simulink model "SML_SSE_RL"  (R2015a)
settings: Solver=ode4  SolverMode=MultiTasking  StartTime=0.0  StopTime=inf  FixedStep=BKIN_STEP_TIME  RelTol=1e-3
StartFcn:
  |  warndlg('Dexterit-E models cannot run under simulation. Please compile your model and run it from within Dexterit-E.');set_param(bdroot,'SimulationCommand','stop')
model workspace (MAT data in the model file):
  col_x = 1
  col_y = 2
  RADIUS_VIS = 3
  COLOR_INIT = 6
  BKIN_STEP_TIME = 0.00025
  E_END_TRIAL = 20
  STROKE_WIDTH = 8
  K_ROBOT_RAMP_TIME = 1
  E_ENABLED_CONTROLLER = 31
  K_TIME_TO_START = 4
  BKIN_KINEMATIC_FRAME_SIZE = 400
  E_NO_EVENT = 0
  STARTTARGET_COL = 1
  MOVE_TIME_COL = 3
  MOVE_XVEL_COL = 4
  MOVE_YVEL_COL = 5
  E_INIT_TRIAL = 1
  E_MOVE_TO_START = 2
  E_AT_START = 4
  E_PASSIVE_HOLD_AT_START = 6
  E_MOVE_TO_END = 8
  COLOR_SELECT = 7
  ACTORPAS_COL = 6
  E_ACTIVE_HOLD_AT_START = 7
  CHANNEL_WIDTH = 1
  WALL_WIDTH = 2
  WALL_STIFFNESS = 3
  WALL_VISCOSITY = 4
  PROBE_COL = 8
  K_TIME_HOLD_START = 5
  E_ENABLE_BUTTONS = 46
  E_DISABLE_BUTTONS = 47
  LABEL_1 = 3
  RESPONSE_AHEAD = 4
  RESPONSE_BEHIND = 5
  B_LABEL_1 = 3
  B_AHEAD = 4
  B_BEHIND = 5
  DYNOREND_COL = 7
  E_REPEAT_TRIAL_FLAG = 35
  END_TARGET_COL = 2
  HEIGHT_VIS = 4
  WIDTH_VIS = 5
  E_TOO_FAST = 11
  E_TOO_SLOW = 12
  PROBE_SHIFT_COL = 9
  K_TIME_PROBE_HOLD = 3
  E_AT_END_TARGET = 10
  K_DELAY_POSTTRIAL = 2
  LABEL_TEXT = 9
  LABEL_HEIGHT = 10
  E_FINISH_MOVE = 49
  E_HIT_PROBE = 48
  E_TEST_1 = 50
  E_JUST_RIGHT = 51
undefined symbols (not defined in the file): slselsubs
libraries: slrtlib x5, KINARM_loads x4, Video x4, General x3, KINARM_general x2, simulink x1, xpcnilib x1
(part 2 of 2)

== matlab function SML_SSE_RL/Force Channel1/Calculate force channel (wall)  ==
  data: target1 input; forces output; target2 input; active_arm input; hand_position input; hand_velocity input; secondary_encoders_used input; loadTable input; enable_forces input
function forces = forceChannel(target1, target2, active_arm, hand_position, hand_velocity, secondary_encoders_used, loadTable, enable_forces)

	persistent lastForcesEnabledValue forceEnableTime clockCycle outsideChannel lastHandPosition;
	
	if isempty(lastForcesEnabledValue), lastForcesEnabledValue = 0;		end
	if isempty(forceEnableTime),        forceEnableTime = 1;			end
	if isempty(clockCycle),				clockCycle = 0;					end
	if isempty(outsideChannel),			outsideChannel = 0;				end
	if isempty(lastHandPosition),		lastHandPosition = zeros(1,2);	end


	%we need to keep track of the time so we can safely ramp up forces when 
	%the trial starts.
	clockCycle = clockCycle + 1;
	if lastForcesEnabledValue == 0 && enable_forces == 1
		forceEnableTime = clockCycle;
	end

	lastForcesEnabledValue = enable_forces;

	%start out assuming we will apply no forces.
	forces = zeros(1, 4);

    channelWidthM = abs((loadTable(1) * 0.01) / 2.0);%get the width of the zero force zone and convert to meters
	wallWidthM = abs(loadTable(2) * 0.01);			%get the width of the wall where forces cut out and convert to meters.
%     if secondary_encoders_used == 0
%         % No secondary encoders
%     	wallStiffness = abs(loadTable(3));				%in N/m
%     	viscosity = -abs(loadTable(4));					%in N/(m/s)
%     else
        % With secondary encoders
    	wallStiffness = abs(loadTable(3));				%in N/m
    	viscosity = -abs(loadTable(4));					%in N/(m/s)
%     end

	xHand=hand_position(1);		%(m)
	yHand=hand_position(2);		%(m)

	%get the target positions and convert them to meters.
	x1 = (-20) * 0.01; 
    %y1 = target1-(loadTable(1)/2)* 0.01;
	y1 = target1* 0.01;   %offset for half of the channel zero force width... puts wall at center of probe instead of at radius.
	x2 = (20) * 0.01;                       %target 2 is projected from target1 and the desired start velocities
	%y2 = target2-(loadTable(1)/2) * 0.01;
    y2 = target2 * 0.01;

	%http://www.codeguru.com/forum/showthread.php?threadid=194400
	%This calculations gives us the distance away from the line we are now.
	distToLine = abs(((x2 - x1)*(y1-yHand)) - ((x1 - xHand)*(y2-y1))) / sqrt( (x2 - x1)^2 + (y2 - y1)^2 );

	HXVEL = hand_velocity(1);
	HYVEL = hand_velocity(2);
	viscosityX = HXVEL * viscosity;
	viscosityY = HYVEL * viscosity;

	%we only ever want to provide a viscous load perpendicular to
	%the force channel. This viscous force will be used to dampen
	%any instability.
	if (x2 == x1) %infinite slope
		viscosityY = 0;	
	elseif (y2 == y1) %0 slope
		viscosityX = 0;
	else
		m = (y2 - y1) / (x2 - x1);
		perpM = -(1/m);	

		%we need to scale the viscous load to only the components
		%that are perpendicular to the line. To do that we find the 
		%projection of the velocity vecotor on a line perpendicular to the
		%force channel
		perpVect = [1 perpM];
		perpUnitVector = perpVect / norm(perpVect);

		%this finds the projection of the vector perpendicular to the channel
		dotProduct = dot([viscosityX viscosityY], perpUnitVector);
		scaledForces = dotProduct * perpUnitVector;

		viscosityX = scaledForces(1);
		viscosityY = scaledForces(2);
	end

	%forces 1,2 are for right arm, 3,4 are for left
	addIdx = 0;
	if active_arm == 2
		addIdx = 2;
	end

	% if we are outside the force wall we need to make sure we don't turn it
	%back on until we are in the channel. Otherwise it's quite jarring to be pulled in.
	if distToLine > (wallWidthM + channelWidthM)
		outsideChannel = 1;
		return
	elseif enable_forces == 0
		return	
	%if we are in the force channel we still need to viscous loads to aid in stability
	%if we are bouncing between the walls. 
	elseif distToLine < channelWidthM 
		outsideChannel = 0; %we're in the channel, so we can turn forces back on if they were off.
		return
	elseif outsideChannel == 1    
		%If we were outside the wall then forces are all off. We only want to turn
		%forces back on if the hand has crossed the line of the force channel, that way
		%you are not pushed into the channel, it only feels like you hit a wall.
		%By looking at the previous hand position and the current hand position
		%we can see if that line segment crosses the channel line, in which case we can
		%turn the forces back on.
		if doLinesIntersect([x1 y1], [x2 y2], [xHand yHand], lastHandPosition) == 1
			outsideChannel = 0;
		else
			return
		end
	end

	distIntoWall = distToLine - channelWidthM;

	if (x2 == x1) %all force wille be in x direction
		y = 0;
		if xHand < x1
			x = distIntoWall;
		else
			x = -distIntoWall;
		end
	elseif (y2 == y1) %all force will be in Y direction
		x = 0;
		if yHand < y1
			y = distIntoWall;
		else
			y = -distIntoWall;
		end	
	else
		%we need to find out how far off the line in X and Y we are in meters so 
		%we can properly convert the wall stiffness in N/m to a force.
		m = (y2 - y1) / (x2 - x1);
		b = y1 - (m * x1);

		perpM = -(1/m);	
		perpB = yHand - (perpM * xHand);

		xIntersect = (b - perpB) / (perpM - m);
		yIntersect = (m * xIntersect) + b;

		%x and y are converted to distances in meters from the center line
		x = xIntersect - xHand;
		y = yIntersect - yHand;

		%take the distances from center and convert to a unit vector,
		%then multiply by the distance to where the forces start
		%this gives us a clean number to use when calculating wall force.
		x = (x / sqrt(x^2 + y^2)) * distIntoWall;
		y = (y / sqrt(x^2 + y^2)) * distIntoWall;
	end

	%we don't want to just shut off the forces, we need to ramp them down
	%somewhat. This finds out how far into the wall we are and allows us
	%to ramp down the forces over the last X% of the wll.
	forceRampDownZoneSizePercent = 0.9; %start ramping down the forces in the last 25% of the wall
	forceMaxEndLocInWallM = forceRampDownZoneSizePercent * wallWidthM;
	distanceIntoWall = distToLine - channelWidthM;
	scaleWallForce = 1; %assume we can run at full calculated wall force

	if distanceIntoWall > forceMaxEndLocInWallM   %we are in the ramp down zone
		distIntoRampDownZone = distanceIntoWall - forceMaxEndLocInWallM;
		rampDownZoneWidth = wallWidthM  - forceMaxEndLocInWallM;
		scaleWallForce = (rampDownZoneWidth - distIntoRampDownZone) / rampDownZoneWidth;
	end

	%within the first 1.5 seconds of the trial we don't wan to jar anyone
	%this ramps the forces up slowly so you get a gentle nudge into
	%the force channel, not a violent jerk.
	timeDelta = clockCycle - forceEnableTime;
	timeScaling = 1;
	if (timeDelta < 1500)
		timeScaling = timeDelta / 1500.0;
	end

	%the final forces will be wall force + viscous.
	forces(addIdx + 1) = (wallStiffness * scaleWallForce * timeScaling * x) + viscosityX;
	forces(addIdx + 2) = (wallStiffness * scaleWallForce  * timeScaling * y) + viscosityY;

	lastHandPosition(1) = xHand;
	lastHandPosition(2) = yHand;
end

function bIntersect = doLinesIntersect(Ap1, Ap2, Bp1, Bp2)
    %This method for finding out if 2 lines segements intersect comes from:
    %http://stackoverflow.com/questions/563198/how-do-you-detect-where-two-line-segments-intersect
   	e = Ap2-Ap1;
    f = Bp2-Bp1;
    p = [-e(2) e(1)];
    h = dot((Ap1 - Bp1), p) / dot (f, p);
    
    if h >=0 && h <= 1
        bIntersect = 1;
    else
        bIntersect = 0;
    end
end

== matlab function SML_SSE_RL/Play Sound/Play sound over and over ==
  data: tone input; output output; Hz500 input; Hz800 input; Hz1200 input
function output = fcn(tone,Hz500,Hz800,Hz1200)
%#codegen

persistent t last_tone_state
if isempty(t), t = 0; end
if isempty(last_tone_state), last_tone_state = 0; end

trigger = last_tone_state ~= tone;
if trigger > 0
    last_tone_state = tone;
end

output = 0;		% default
if t == 0 && trigger > 0
	% start the playing of the sound.
	t = t + 1;
end

if tone == 1
    data = Hz500;
elseif tone == 2
    data = Hz800;
elseif tone == 3
    data = Hz1200;
else 
    t = 0;
    data = 0;
end

if t > 0
	output = data(t);
	if t == length(data)
		t = 0;
	else
		t = t + 1;
	end
end

== matlab function SML_SSE_RL/Force Channel/Calculate force channel ==
  data: target1 input; forces output; target2 input; xIdx input; yIdx input; active_arm input; hand_position input; hand_velocity input; secondary_encoders_used input; loadTable input; enable_forces input
function forces = forceChannel(target1, target2, xIdx, yIdx, active_arm, hand_position, hand_velocity, secondary_encoders_used, loadTable, enable_forces)

	persistent lastForcesEnabledValue forceEnableTime clockCycle outsideChannel lastHandPosition;
	
	if isempty(lastForcesEnabledValue), lastForcesEnabledValue = 0;		end
	if isempty(forceEnableTime),        forceEnableTime = 1;			end
	if isempty(clockCycle),				clockCycle = 0;					end
	if isempty(outsideChannel),			outsideChannel = 0;				end
	if isempty(lastHandPosition),		lastHandPosition = zeros(1,2);	end


	%we need to keep track of the time so we can safely ramp up forces when 
	%the trial starts.
	clockCycle = clockCycle + 1;
	if lastForcesEnabledValue == 0 && enable_forces == 1
		forceEnableTime = clockCycle;
	end

	lastForcesEnabledValue = enable_forces;

	%start out assuming we will apply no forces.
	forces = zeros(1, 4);

    channelWidthM = abs((loadTable(1) * 0.01) / 2.0);%get the width of the zero force zone and convert to meters
	wallWidthM = abs(loadTable(2) * 0.01);			%get the width of the wall where forces cut out and convert to meters.
%     if secondary_encoders_used == 0
%         % No secondary encoders
%     	wallStiffness = abs(loadTable(3));				%in N/m
%     	viscosity = -abs(loadTable(4));					%in N/(m/s)
%     else
        % With secondary encoders
    	wallStiffness = abs(loadTable(3));				%in N/m
    	viscosity = -abs(loadTable(4));					%in N/(m/s)
%     end

	xHand=hand_position(1);		%(m)
	yHand=hand_position(2);		%(m)

	%get the target positions and convert them to meters.
	x1 = target1(xIdx) * 0.01;
	y1 = target1(yIdx) * 0.01;
	x2 = target2(1) * 0.01;  %target 2 is projected from target1 and the desired start velocities
	y2 = target2(2) * 0.01;

	%http://www.codeguru.com/forum/showthread.php?threadid=194400
	%This calculations gives us the distance away from the line we are now.
	distToLine = abs(((x2 - x1)*(y1-yHand)) - ((x1 - xHand)*(y2-y1))) / sqrt( (x2 - x1)^2 + (y2 - y1)^2 );

	HXVEL = hand_velocity(1);
	HYVEL = hand_velocity(2);
	viscosityX = HXVEL * viscosity;
	viscosityY = HYVEL * viscosity;

	%we only ever want to provide a viscous load perpendicular to
	%the force channel. This viscous force will be used to dampen
	%any instability.
	if (x2 == x1) %infinite slope
		viscosityY = 0;	
	elseif (y2 == y1) %0 slope
		viscosityX = 0;
	else
		m = (y2 - y1) / (x2 - x1);
		perpM = -(1/m);	

		%we need to scale the viscous load to only the components
		%that are perpendicular to the line. To do that we find the 
		%projection of the velocity vecotor on a line perpendicular to the
		%force channel
		perpVect = [1 perpM];
		perpUnitVector = perpVect / norm(perpVect);

		%this finds the projection of the vector perpendicular to the channel
		dotProduct = dot([viscosityX viscosityY], perpUnitVector);
		scaledForces = dotProduct * perpUnitVector;

		viscosityX = scaledForces(1);
		viscosityY = scaledForces(2);
	end

	%forces 1,2 are for right arm, 3,4 are for left
	addIdx = 0;
	if active_arm == 2
		addIdx = 2;
	end

	% if we are outside the force wall we need to make sure we don't turn it
	%back on until we are in the channel. Otherwise it's quite jarring to be pulled in.
	if distToLine > (wallWidthM + channelWidthM)
		outsideChannel = 1;
		return
	elseif enable_forces == 0
		return	
	%if we are in the force channel we still need to viscous loads to aid in stability
	%if we are bouncing between the walls. 
	elseif distToLine < channelWidthM 
		outsideChannel = 0; %we're in the channel, so we can turn forces back on if they were off.
		return
	elseif outsideChannel == 1    
		%If we were outside the wall then forces are all off. We only want to turn
		%forces back on if the hand has crossed the line of the force channel, that way
		%you are not pushed into the channel, it only feels like you hit a wall.
		%By looking at the previous hand position and the current hand position
		%we can see if that line segment crosses the channel line, in which case we can
		%turn the forces back on.
		if doLinesIntersect([x1 y1], [x2 y2], [xHand yHand], lastHandPosition) == 1
			outsideChannel = 0;
		else
			return
		end
	end

	distIntoWall = distToLine - channelWidthM;

	if (x2 == x1) %all force wille be in x direction
		y = 0;
		if xHand < x1
			x = distIntoWall;
		else
			x = -distIntoWall;
		end
	elseif (y2 == y1) %all force will be in Y direction
		x = 0;
		if yHand < y1
			y = distIntoWall;
		else
			y = -distIntoWall;
		end	
	else
		%we need to find out how far off the line in X and Y we are in meters so 
		%we can properly convert the wall stiffness in N/m to a force.
		m = (y2 - y1) / (x2 - x1);
		b = y1 - (m * x1);

		perpM = -(1/m);	
		perpB = yHand - (perpM * xHand);

		xIntersect = (b - perpB) / (perpM - m);
		yIntersect = (m * xIntersect) + b;

		%x and y are converted to distances in meters from the center line
		x = xIntersect - xHand;
		y = yIntersect - yHand;

		%take the distances from center and convert to a unit vector,
		%then multiply by the distance to where the forces start
		%this gives us a clean number to use when calculating wall force.
		x = (x / sqrt(x^2 + y^2)) * distIntoWall;
		y = (y / sqrt(x^2 + y^2)) * distIntoWall;
	end

	%we don't want to just shut off the forces, we need to ramp them down
	%somewhat. This finds out how far into the wall we are and allows us
	%to ramp down the forces over the last X% of the wll.
	forceRampDownZoneSizePercent = 0.9; %start ramping down the forces in the last 25% of the wall
	forceMaxEndLocInWallM = forceRampDownZoneSizePercent * wallWidthM;
	distanceIntoWall = distToLine - channelWidthM;
	scaleWallForce = 1; %assume we can run at full calculated wall force

	if distanceIntoWall > forceMaxEndLocInWallM   %we are in the ramp down zone
		distIntoRampDownZone = distanceIntoWall - forceMaxEndLocInWallM;
		rampDownZoneWidth = wallWidthM  - forceMaxEndLocInWallM;
		scaleWallForce = (rampDownZoneWidth - distIntoRampDownZone) / rampDownZoneWidth;
	end

	%within the first 1.5 seconds of the trial we don't wan to jar anyone
	%this ramps the forces up slowly so you get a gentle nudge into
	%the force channel, not a violent jerk.
	timeDelta = clockCycle - forceEnableTime;
	timeScaling = 1;
	if (timeDelta < 1500)
		timeScaling = timeDelta / 1500.0;
	end

	%the final forces will be wall force + viscous.
	forces(addIdx + 1) = (wallStiffness * scaleWallForce * timeScaling * x) + viscosityX;
	forces(addIdx + 2) = (wallStiffness * scaleWallForce  * timeScaling * y) + viscosityY;

	lastHandPosition(1) = xHand;
	lastHandPosition(2) = yHand;
end

function bIntersect = doLinesIntersect(Ap1, Ap2, Bp1, Bp2)
    %This method for finding out if 2 lines segements intersect comes from:
    %http://stackoverflow.com/questions/563198/how-do-you-detect-where-two-line-segments-intersect
   	e = Ap2-Ap1;
    f = Bp2-Bp1;
    p = [-e(2) e(1)];
    h = dot((Ap1 - Bp1), p) / dot (f, p);
    
    if h >=0 && h <= 1
        bIntersect = 1;
    else
        bIntersect = 0;
    end
end

== stateflow chart SML_SSE_RL/Trial Control ==
  note: THINGS TO NOTE:
      | Old MATLAB random shift function left in case needed in future
      | K denotes taskwide parameters
      | E denotes event codes
  state init/
    ramp_time = TaskwideParams[K_ROBOT_RAMP_TIME];
    enable_controller = 0;
    tone = 0;
    EndPos[1] = 0;
    EndPos[2] = 0;
    ForceScale = 0;
    ForceChannelState = 0; //turn off the force channel
    forceWallState = 0; //turn off force wall
    trajtype = 0;  //set to 1 to be constant velocity, set to 0 to be bezier
    logging_enable = 0;
    probeY = 100;
    initializeCursor = 1;
  state Main/
    state HoldAtStart/
      event_code=E_AT_START;
      curHandPosY = CurHandPos[2];
      endOfTrial = 1;
      //reset all the move and shift parameters
      StartTarget = Trial_Protocol[STARTTARGET_COL];
      EndTarget = Trial_Protocol[END_TARGET_COL];
      targetWall = Target_Table[Trial_Protocol[PROBE_COL]][2]; %y value of center of probe target
      StartPos[1] = Target_Table[StartTarget][1];
      StartPos[2] = Target_Table[StartTarget][2];
      MoveVel[1] = 0;
      MoveVel[2] = 0;
      MoveTime = 0;
      TargetShiftTime = 0;
      ShowTime =0;
      logging_enable = 1;
      // Probe Targets
      //Probe = Trial_Protocol[PROBE_COL];
      //randShift = pickRand(11);
      randShift = Trial_Protocol[PROBE_SHIFT_COL];
      probeY = Target_Table[Trial_Protocol[PROBE_COL]][2];
      exit:
      endOfTrial = 0;
    state InitTrial/
      event_code=E_INIT_TRIAL;
      StartPos[1] = CurHandPos[1];
      StartPos[2] = CurHandPos[2];
      EndPos[1] = Target_Table[Trial_Protocol[STARTTARGET_COL]][1];
      EndPos[2] = Target_Table[Trial_Protocol[STARTTARGET_COL]][2];
      MoveTime = TaskwideParams[K_TIME_TO_START];
      //randShift = 6; //corresponding zero value from randomizing in Stateflow and not Dex
      enable_controller = 0;
      t_step = 0;
      tone = 0;
      logging_enable = 0;
      startCursorFeedback = 0;
      Repeat_Trial_Flag = 0;
      forceWallState = 0;
      tickCountSnow = 0;
    state MoveArmToStartTarget/
      event_code=E_MOVE_TO_START;
      enable_controller = 1;
      trajtype = 0;  //set to 1 to be constant velocity, set to 0 to be bezier
      ForceChannelState = 0; //turn off the force channel
      ForceScale = 1; //let the automatic ramp take care of turning the forces on
      //increment t_step on each clock cycle
      during:
      on e_clk: t_step = t_step + (1/ (MoveTime/1000 * 1000));
      HandVel = sqrt(HandVelocity[1]^2 + HandVelocity[2]^2);
      exit:
      Probe_State = 0;
    state Selections/
      AorP = Trial_Protocol[ACTORPAS_COL];
      DorE = Trial_Protocol[DYNOREND_COL];
    state SetActiveMoveParameters/
      startCursorFeedback = 0; //turn off hand position
      //set up the target shift parameters
      MoveTime = Trial_Protocol[MOVE_TIME_COL];
      MoveVel[1] = Trial_Protocol[MOVE_XVEL_COL];
      MoveVel[2] = Trial_Protocol[MOVE_YVEL_COL];
      EndPos[1] = Target_Table[END_TARGET_COL][1];
      EndPos[2] = Target_Table[END_TARGET_COL][2];
      vthreshMax = 0;
      vthreshUB = 0.12; //eliminate jerkiness cm/s
      movdir = atan2(MoveVel[2],MoveVel[1]) * 180/pi;
      trajtype = 0;  //set to 1 to be constant velocity, set to 0 to be bezier
      //turn on the force channel
      ForceChannelState = 1; //turn on the force channel
    state PassiveHoldAtStart1/
      event_code=E_PASSIVE_HOLD_AT_START;
      ForceScale = 1;
      startCursorFeedback = 1;
      enable_controller = 1;
      t_step = 0;
      tickCount = TaskwideParams[K_TIME_HOLD_START];
      //movement parameters
      trajtype = 1;  //set to 1 to be constant velocity, set to 0 to be bezier
      MoveVel[1] = Trial_Protocol[MOVE_XVEL_COL];
      MoveVel[2] = Trial_Protocol[MOVE_YVEL_COL];
      EndPos[1] = Target_Table[Trial_Protocol[END_TARGET_COL]][1];
      EndPos[2] = Target_Table[Trial_Protocol[END_TARGET_COL]][2]
      MoveTime = Trial_Protocol[MOVE_TIME_COL];
      movdir = atan2(MoveVel[2],MoveVel[1]) * 180/pi;
      exit:
      tone = 1;
      startCursorFeedback = 0;
    state ActiveHoldAtStart/
      event_code=E_ACTIVE_HOLD_AT_START;
      startCursorFeedback = 1;
      enable_controller = 1;
      t_step = 0;
      tickCount = TaskwideParams[K_TIME_HOLD_START] - 50;
      //next hold is 50 ms to ensure no skipping
      exit:
      enable_controller = 0;
      ForceScale = 0;
      startCursorFeedback = 0;
      tickCount = 0;
    state MoveArm/
      event_code=E_MOVE_TO_END;
      tickCount = 0; //initialize counter
      during:
      curHandPosY = CurHandPos[2];
      on e_clk: t_step = t_step + (1/ (MoveTime/1000 * 1000));
      exit:
      //ForceScale = 0.4; //smooth out hand catch
    state DuringEndpointMovement/
      tone = 1;
      event_code=E_MOVE_TO_END;
      tickCountSnow = 4000;	//satisfy Dynamic criteria since not needed in this part
      tickCountSnowA = 0;
      tickCountSnowB = 0;
      probeY = Target_Table[Trial_Protocol[PROBE_COL]][2]-0.5;
      during:
      on e_clk: tickCountSnowA++;
      curHandPosY = CurHandPos[2];
      HandVel = sqrt(HandVelocity[1]^2 + HandVelocity[2]^2);
      vthreshMax = vthreshMax || (HandVel > vthreshUB); //true if you ever exceed UB
      exit:
      ForceChannelState = 0; //turn off the force channel
      StartPos[1] = CurHandPos[1];
      StartPos[2] = CurHandPos[2];
      EndPos[1] = CurHandPos[1];
      EndPos[2] = Target_Table[Trial_Protocol[PROBE_COL]][2];
    state DuringDynamicMovement/
      event_code=E_MOVE_TO_END;
      tickCountSnow = 0;
      //vthreshUB = 0.08;
      //vthreshLB = 0.02;
      vAVGp1 = 0.05;
      vAVGp2 = 0.05;
      tone = 1;
      during:
      on e_clk: tickCountSnow++;
      HandVel = sqrt(HandVelocity[1]^2 + HandVelocity[2]^2);
      vthreshMax = vthreshMax || (HandVel > vthreshUB); //true if you ever exceed UB
      curHandPosY = CurHandPos[2];
      exit:
      ForceChannelState = 0;
    state OnceHitProbe1/
      entry:
      event_code=E_HIT_PROBE;
      tickCount = TaskwideParams[K_TIME_PROBE_HOLD];
      during:
      curHandPosY = CurHandPos[2];
      exit:
      tickCountSnow = 0; //just to be sure
    state InProbe/
      entry:
      event_code=E_HIT_PROBE;
      enable_controller = 1;
      trajtype = 0;  //set to 1 to be constant velocity, set to 0 to be bezier
      ForceScale = .2; //let the automatic ramp take care of turning the forces on
      tickCount = TaskwideParams[K_TIME_PROBE_HOLD];
      during:
      curHandPosY = CurHandPos[2];
      exit:
      StartPos[1] = Target_Table[StartTarget][1]; //important to change these so force channel doesn't change
      StartPos[2] = Target_Table[StartTarget][2];
      EndPos[1] = Target_Table[END_TARGET_COL][1];
      EndPos[2] = Target_Table[END_TARGET_COL][2];
      enable_controller = 0;
      tickCount = 0;
      ForceScale = 0;
    state FinishPassiveMove/
      event_code=E_FINISH_MOVE;
      during:
      on e_clk: t_step = t_step + (1/ (MoveTime/1000 * 1000)); //Continue movement
      exit:
      //ForceScale = 0.5; //smooth out the hand catch a little bit
    state StopActiveMovement/
      entry:
      event_code = E_AT_END_TARGET
      //if we have moved long enough, catch the hand to stop it from moving
      enable_controller = 1;  //turn on the position controller to catch the hand
      trajtype = 0;  //set to 1 to be constant velocity, set to 0 to be bezier
      StartPos[1] = CurHandPos[1];
      StartPos[2] = CurHandPos[2];
      ForceScale = 1;
    state MoveToEnd/
      entry:
      event_code=E_FINISH_MOVE;
      ForceChannelState = 1;
      during:
      on e_clk: tickCountSnowB++;
      curHandPosY = CurHandPos[2];
      HandVel = sqrt(HandVelocity[1]^2 + HandVelocity[2]^2);
      //true if you ever exceed LB (bottom)
      exit:
      ForceChannelState = 0;
      //calculations for ENDPOINT average velocity for phase 1 and 2
      vAVGp1 = ((Target_Table[Trial_Protocol[PROBE_COL]][2]-Target_Table[StartTarget][2])/100)/(tickCountSnowA/1000);
      vAVGp2 = ((Target_Table[EndTarget][2]-Target_Table[Trial_Protocol[PROBE_COL]][2])/100)/(tickCountSnowB/1000);
    state TestState/
      event_code=E_TEST_1;
    state HoldAtEnd/
      event_code=E_AT_END_TARGET;
      t_step = 1;
      trajtype = 0;
    state WaitForResponse/
      event_code = E_ENABLE_BUTTONS;
    state JustRight/
      event_code = E_JUST_RIGHT;
    state Disable_Buttons/
      event_code = E_DISABLE_BUTTONS;
    state TooSlow/
      event_code = E_TOO_SLOW
      Probe_State = 1;
      Probe = 3; //3rd row
    state TooFast/
      event_code = E_TOO_FAST
      Probe_State = 1;
      Probe = 4;
    state MissTarget1/ [commented out]
      Repeat_Trial_Flag = 1;
      event_code = E_REPEAT_TRIAL_FLAG
      //The speed of the reach was not acceptable
    state EndOfTrial/
      event_code = E_END_TRIAL;
      StartPos[1] = CurHandPos[1];
      StartPos[2] = CurHandPos[2];
      t_step = 0;
      tickCount =Trial_Protocol[K_DELAY_POSTTRIAL];
      tone = 0;
    state MissTarget/
      Repeat_Trial_Flag = 1;
      event_code = E_REPEAT_TRIAL_FLAG
      //This was used for different logic and/should not be
      //possible unless probe is defined before endpoint
    InitTrial -> MoveArmToStartTarget : after(50,e_clk)
    MoveArmToStartTarget -> HoldAtStart : // t done incrementing
        | [(t_step >= 1)]/
        | t_step = 1;
    HoldAtStart -> (junction 813) : after(50, e_clk)
    (junction 813) -> Selections
    Selections -> ActiveHoldAtStart [order 2] : //active condition
        | [AorP > 0]
    Selections -> PassiveHoldAtStart1 [order 1] : //passive condition
        | [AorP <= 0]
    ActiveHoldAtStart -> SetActiveMoveParameters : after(tickCount,e_clk)
    PassiveHoldAtStart1 -> MoveArm : after(tickCount,e_clk)
    SetActiveMoveParameters -> (junction 774) : after(50,e_clk)
        | //this allows time for force channel to switch on
    (junction 774) -> DuringDynamicMovement [order 2] : [DorE == 1] //DYNAMIC
    (junction 774) -> DuringEndpointMovement [order 1] : [DorE == 0] //ENDPOINT
    MoveArm -> (junction 811) [order 1] : [t_step >=1 && DorE == 1]
    (junction 811) -> HoldAtEnd
    MoveArm -> (junction 779) [order 3] : [(t_step >= 1) && (DorE == 0)]
    (junction 779) -> MissTarget
    MoveArm -> OnceHitProbe1 [order 2] : //ENDPOINT
        | [(CurHandPos[2] >= Target_Table[Trial_Protocol[PROBE_COL]][2] && DorE ==0)]
    DuringEndpointMovement -> InProbe : [(CurHandPos[2] >= Target_Table[Trial_Protocol[PROBE_COL]][2]-0.5)]
    DuringDynamicMovement -> StopActiveMovement : [(CurHandPos[2] >= Target_Table[EndTarget][2])]
    OnceHitProbe1 -> FinishPassiveMove : //wait time in probe specified in GUI
        | after(tickCount, e_clk)
    InProbe -> MoveToEnd : after(tickCount,e_clk)
    FinishPassiveMove -> HoldAtEnd : // t done incrementing
        | [(t_step >= 1)]/
        | t_step = 1;
    MoveToEnd -> StopActiveMovement : [(CurHandPos[2] >= Target_Table[EndTarget][2])]
    StopActiveMovement -> TestState : after(50,e_clk)
    TestState -> (junction 675)
    HoldAtEnd -> WaitForResponse : after(50, e_clk)
    JustRight -> WaitForResponse
    (junction 675) -> JustRight [order 3]
    (junction 675) -> TooSlow [order 1] : [(tickCountSnow>=5000)||(vAVGp1 <= 0.02 || vAVGp2 <= 0.02)]
    (junction 796) -> WaitForResponse : after(50,e_clk)
    (junction 675) -> TooFast [order 2] : [tickCountSnow<3333 ||(vAVGp1 > 0.06 || vAVGp2 > 0.06)]
    WaitForResponse -> Disable_Buttons : [after(1,e_clk) && (ButtonInput == 1)]/
    Disable_Buttons -> EndOfTrial : after(50,e_clk)
    TooSlow -> (junction 796)
    TooFast -> (junction 796)
    MissTarget1 -> ? [commented out] : after(50, e_clk)
    MissTarget -> EndOfTrial : after(50, e_clk)
  state Inter_Trial_State1/
    //reset the event code, and send the
    //e_Trial_End Stateflow event to indicate that the trial is over.
    event_code = 0;
    tickCount = 100;
    e_Trial_End;
  state RobotRampDown/
    enable_controller = 0;
    ramp_time = 2000;
  (default) -> init
  init -> InitTrial
  (junction 817) -> InitTrial
  Inter_Trial_State1 -> (junction 817) : // has a a specified period of
      | // time occured?
      | after(tickCount, e_clk)
  Main -> RobotRampDown : e_ExitTrialNow/
      | tickCount = 1;
      | // e_ExitTrialNow event occurs if the
      | // Dex pause is pressed by the operator
  RobotRampDown -> Inter_Trial_State1 : after(ramp_time,e_clk)
  (junction 815) -> Inter_Trial_State1
  EndOfTrial -> (junction 815) : after(50, e_clk)
  data: randShift function_output double; upperBound function_input double; data local double; logging_enable output double; event_code output uint16 [0..] =0; AorP output double; DorE output double size=1; movdir output double; enable_controller output double; ForceScale output double [0..1]; tickCount local double; Trial_Protocol input double; HandInTargetProbe input; TaskwideParams input double; HandVelocity input double; t_step output double size=1; HandVel local double; StartPos output double size=[1 2]; MoveVel output double size=[1 2]; EndPos output double size=[1 2]; trajtype output double size=1; ForceChannelState output double; StartTarget output double; forceWallState output double size=1; targetWall output double; Target_Table input double size=[64 25]; CurHandPos input double size=[1 2]; MoveTime local double; ShowTime local double; TargetShiftTime local double; pi parameter double =3.141592653589793; vthreshMax local double; vthreshMin local double; ramp_time local double; vthreshUB local double; vthreshLB local double; Probe output double size=1; Probe_State output double size=1; tickCountSnow local double size=1; ButtonInput input; randShift output double; probeY output double; curHandPosY output double; endOfTrial output double; initializeCursor output double; startCursorFeedback output size=1; tone output double size=1; Repeat_Trial_Flag output double size=1; vthreshLB2 local double; vthreshMin2 local double; tickCountSnowA local double; tickCountSnowB local double; vAVGp1 local double; vAVGp2 local double; EndTarget local double
  events: e_clk input RISING_EDGE_EVENT; e_ExitTrialNow input EITHER_EDGE_EVENT; e_Trial_End output EITHER_EDGE_EVENT
  function randShift = pickRand(upperBound):
    | function randShift = pickRand(upperBound)
    | randShift = randi(upperBound)
    | end

== matlab function SML_SSE_RL/MakeTraj/pos_velramp ==
  data: startxy input size=[1 2]; handvel input; t input; desiredPos output size=[1 2]; VCODE input; VCODE_mod output
function [desiredPos,VCODE_mod] = fcn(startxy,handvel,t,VCODE)
%#codegen

%xy position in cm, velocity in m/s

startxy = startxy/100; %convert to meters

xvel = handvel(1)*10;
yvel = handvel(2)*10;

VCODE_mod = VCODE;

%clip t just in case!
if t < 0
    t = 0;
elseif t > 1;
    t = 1;
end

%we will spend the first 10% of the movement accelerating and the last 10%
%of the movement decelerating. we will use a trapezoidal profile for
%simplicity

xshift = 0;
yshift = 0;

if t < 0.1
    
    %xshift = 0.5*xvel*t;
    %yshift = 0.5*yvel*t;
    xshift = xvel/(.2)*t^2;
    yshift = yvel/(.2)*t^2;
    
elseif t < 0.9

    %xshift = 0.5*xvel*0.1 + (t-0.1)*xvel;
    %yshift = 0.5*yvel*0.1 + (t-0.1)*yvel;
    xshift = xvel/(.2)*0.1^2 + (t-0.1)*xvel;
    yshift = yvel/(.2)*0.1^2 + (t-0.1)*yvel;
    
elseif t <= 1

    %xshift = 0.5*xvel*0.1 + (t-0.1)*xvel + 0.5*xvel*(t-0.9);
    %yshift = 0.5*yvel*0.1 + (t-0.1)*yvel + 0.5*yvel*(t-0.9);
    xshift = xvel/(.2)*0.1^2 + (t-0.1)*xvel + xvel/(0.2)*(t-0.9)^2;
    yshift = yvel/(.2)*0.1^2 + (t-0.1)*yvel + yvel/(0.2)*(t-0.9)^2;
    
end

xpos = startxy(1)+xshift;
ypos = startxy(2)+yshift;

desiredPos = [xpos ypos];

VCODE_mod(1,3) = desiredPos(1); %convert to meters
VCODE_mod(1,4) = desiredPos(2); %convert to meters

== stateflow chart SML_SSE_RL/Subsystem2/Chart ==
  state EnableState/
    state AutoMoveToPos/
      //smoothly creates a trajectory to get the hand to a point eventually
      state MovingToDesiredXY/
        tickCount = TaskwideParams[K_TIME_TO_START];
        state = 11;
        tick = 0;
        during:
        on e_clk: tick++;
        // the trajectory velocity will have a bell shaped profile
        trajectory_shape = tick/tickCount-sin(2*pi*tick/tickCount)/(2*pi);
        virtual_pos[1] = StartPos[1] + (TgtPos[1] - StartPos[1]) * trajectory_shape;
        virtual_pos[2] = StartPos[2] + (TgtPos[2] - StartPos[2]) * trajectory_shape;
      state GetDesiredXY/
        //grab the current desired pos in case it changes
        TgtPos[1] = DesiredPos[1];
        TgtPos[2] = DesiredPos[2];
        StartPos[1] = HandPos[1];
        StartPos[2] = HandPos[2];
        updatepos = 0;
        state = 10;
      state HoldAtDesiredXY/
        //pause until something changes
        state = 12;
        updatepos = 0;
        during:
        on e_clk: updatepos = ( (abs(TgtPos[1]-DesiredPos[1]) > 0.01) || (abs(TgtPos[2]-DesiredPos[2]) > 0.01) )
      GetDesiredXY -> MovingToDesiredXY : after(1, e_clk)
      HoldAtDesiredXY -> GetDesiredXY : [updatepos == 1 && MovOnTraj == 0]
      MovingToDesiredXY -> HoldAtDesiredXY : after(tickCount, e_clk)/
    state MoveAlongTraj/
      //take a step along a trajectory specified externally
      state GetDesiredXY_Traj/
        TgtPos[1] = DesiredPos[1];
        TgtPos[2] = DesiredPos[2];
        StartPos[1] = HandPos[1];
        StartPos[2] = HandPos[2];
        state = 21;
        //movIsSafe = ( (abs(TgtPos[1]-HandPos[1]) < 0.02) || (abs(TgtPos[2]-HandPos[2]) < 0.02) );
        movIsSafe = 1;
      state MovAlongTraj/
        state = 22;
        virtual_pos[1] = DesiredPos[1];
        virtual_pos[2] = DesiredPos[2];
      GetDesiredXY_Traj -> MovAlongTraj [order 2] : [movIsSafe == 1]
      MovAlongTraj -> GetDesiredXY_Traj
    (junction 15) -> GetDesiredXY [order 1] : [MovOnTraj == 0]
    (junction 15) -> GetDesiredXY_Traj [order 2] : [MovOnTraj == 1]
    MoveAlongTraj -> GetDesiredXY : [MovOnTraj == 0]
    GetDesiredXY_Traj -> GetDesiredXY [order 1] : [movIsSafe == 0]
    AutoMoveToPos -> GetDesiredXY_Traj : [MovOnTraj == 1]
  state RampUp/
    //ramp up the force scale to 1
    CurHandPos[1] = HandPos[1];
    CurHandPos[2] = HandPos[2];
    virtual_pos[1] = HandPos[1];
    virtual_pos[2] = HandPos[2];
    state = 2;
    force_scale = 0;
    during:
    on e_clk: force_scale += scale_increment;
  state Init/
    ramp_time = TaskwideParams[K_ROBOT_RAMP_TIME];
    scale_increment = 1/ramp_time;
    force_scale = 0;
    state = 1;
    during:
    CurHandPos[1] = HandPos[1];
    CurHandPos[2] = HandPos[2];
  state ResetController/
    reset_controller;
  state RampDown/
    //ramp down the force scale to 1
    CurHandPos[1] = HandPos[1];
    CurHandPos[2] = HandPos[2];
    virtual_pos[1] = CurHandPos[1];
    virtual_pos[2] = CurHandPos[2];
    state = 30
    during:
    on e_clk: force_scale -= scale_increment;
  (default) -> Init
  Init -> ResetController : //if controller becomes enabled
      | [enable_controller == 1]/
      | force_scale = 0;
  ResetController -> RampUp
  RampUp -> (junction 15) [order 2] : [force_scale >= 1]/
      | force_scale = 1;
  RampDown -> Init [order 2] : [force_scale <0]/
      | force_scale = 0;
  RampDown -> RampUp [order 1] : [enable_controller == 1]
      | //if the controller is enabled
  RampUp -> RampDown [order 1] : [enable_controller == 0]
      | //if the controller gets shut off
  EnableState -> RampDown : [enable_controller == 0]
  data: enable_controller input double; DesiredPos input; HandPos input; TaskwideParams input; force_scale output double; virtual_pos output double size=2; tickCount local double; StartPos local double size=2; TgtPos local double size=2; updatepos local boolean; MovOnTraj input double; CurHandPos local double size=2; ramp_time local double; scale_increment local double; tick local double; trajectory_shape local double; movIsSafe local boolean; pi constant double =3.14159265358979; state output double
  events: e_clk input EITHER_EDGE_EVENT; reset_controller output EITHER_EDGE_EVENT

== matlab function SML_SSE_RL/Subsystem2/MATLAB Function ==
  data: pos input; VCODE_MOD output; VCODE input
function VCODE_MOD = fcn(pos,VCODE)
%#codegen

VCODE_MOD = VCODE;

VCODE_MOD(3) = pos(1);
VCODE_MOD(4) = pos(2);

== stateflow chart SML_SSE_RL/Shifted Feedback /Chart ==
  note: *ALL TICKS ON GLOABAL COUNTER ARE HALVED FOR SOME REASON... MULTIPLY ALL NUMBERS BY TWO TO GET AROUND*
  state Main/
    state CountAndShowHand/
      entry:
      showHand = 1;
      during:
      on e_clk: tickCountC++;
    state StartTrial/
      tickCountC = 0;
      showHand = 0;
    state DynorEnd/
      wait = 600*2; //600ms
    state TurnOffHandFeedback/
      showHand = 0;
    DynorEnd -> CountAndShowHand [order 1] : [DorE == 1]
    StartTrial -> DynorEnd : //if controller becomes enabled
        | [enable_controllerC == 1]
    DynorEnd -> CountAndShowHand [order 2] : after(wait,e_clk)
        | //in endpoint, wait 600ms
        | //before showing cursor
    TurnOffHandFeedback -> StartTrial : [endOfTrial == 1]
    CountAndShowHand -> TurnOffHandFeedback : [tickCountC >=600*2]
  state Init/
  (default) -> Init : [initializeCursor == 1]
  Init -> StartTrial
  data: showHand output double; tickCountC local double; endOfTrial input double; DorE input; enable_controllerC input double; wait local double; initializeCursor input
  events: e_clk input EITHER_EDGE_EVENT

== matlab function SML_SSE_RL/MakeTraj/PassThrough ==
  data: startxy input; pos output; VCODE input; VCODE_mod output
function [pos,VCODE_mod] = fcn(startxy,VCODE)
%#codegen

%this function passes the input directly to the output. 
%NOTE, THIS CAN BE VERY DANGEROUS TO ENGAGE, AS IT DOES NOT SHAPE THE
% OUTPUT "NICELY" BEFORE SENDING IT TO THE POSITION CONTROLLER 

VCODE_mod = VCODE;

pos = startxy/100;  %convert cm to m

VCODE_mod(1,3) = pos(1);
VCODE_mod(1,4) = pos(2);

== matlab function SML_SSE_RL/Hand_Feedback/FeedFwdArm ==
  settings: fimath=|
      | fimath(...
      | 'RoundMode', 'floor',...
      | 'OverflowMode', 'wrap',...
      | 'ProductMode', 'KeepLSB', 'ProductWordLength', 32,...
      | 'SumMode', 'KeepLSB', 'SumWordLength', 32,...
      | 'CastBeforeSum', false)
  data: KINARMdata input; VCODES_in input; VCODES_out output; fdbk_stts_mdl input; block_settings input
function VCODES_out  = fcn(KINARMdata,VCODES_in,fdbk_stts_mdl, block_settings)
%
% This function creates the VCODEs for the hand position feedback for both
% hands.  Various options in the Mask of the Simulink block in which this
% embedded Matlab file sits, allow the user to specify how often
% the hand feedback is updated as well as the source of the style and status
% of the hand feedback.  
%
% block_settings is the value chosen by the user in the Mask for parent Simulink
% block.  Note: that even if the block is wired up to accept Task Program 
% control of hand feedback style and status, this embedded Matlab file allows
% the GUI to over-ride those settings.  However, if the GUI requests that
% the parent block use Task Program control for the style and/or status when
% it has not been programmed in, then this embedded Matlab file handles this
% appropriately and ignore the request for Task Program control.  
%
% block_settings=1 -- parent block does not have any Task Program control over style or status
% block_settings=2 -- parent block has Task Program control over status only
% block_settings=3 -- parent block has Task Program control over both style and status
%
% fdbk_stts_mdl (only potentially used if block_settings=2) 
% fdbk_stts_mdl=0 -- neither hand on
% fdbk_stts_mdl=1 -- dominant hand on
% fdbk_stts_mdl=2 -- non-dominant hand on
% fdbk_stts_mdl=3 -- both hands on
%
% VCODES (only potentially used if block_settings=3) 
% VCODES for dominant and non-dominant, input to parent block 


dominant_arm=KINARMdata(3,1);
feedfwd=KINARMdata(3,2);				%amount of feedforward extrapolation for hand position(s)
fdbk_stts_GUI=KINARMdata(3,3);			%status of hand feedback requested from GUI
fdbk_src_GUI=KINARMdata(3,4);			%source of hand feedback style requested from GUI
fdbk_clr_GUI=KINARMdata(3,5);			%colour of hand feedback required by GUI
fdbk_radius_GUI=KINARMdata(3,6);		%radius of hand feedback required by GUI


%----------------Feedback Style ----------------
% IF GUI asks for feedback style from Task Program (fdbk_src_GUI==0)
% AND if Task Program has been chosen to supply feedback style (block_settings==3)
% AND if Task Program actually supplies appropriate feedback styles (size(VCODES_in,2)==70)
if fdbk_src_GUI==0 && block_settings==3 && size(VCODES_in,2)==70
    VCODES=VCODES_in;
else
    VCODES=zeros(2,70);						%set default
	VCODES(:,1)=1;							%target_type of circle
	VCODES(:,5)=fdbk_clr_GUI;				%fill colour as specified by GUI
	VCODES(:,6)=fdbk_clr_GUI;				%stroke colour same as fill colour
	VCODES(:,7)=0;							%no stroke width
    VCODES(:,9)=100.0;                      %100% opacity
	VCODES(:,10)=fdbk_radius_GUI;			%radius (m) as specified by GUI
end

%----------------Feedback Status ----------------
%feedback status from GUI sets the default to be used
feedback_status=fdbk_stts_GUI;


if fdbk_stts_GUI==4				%if GUI has requested Task Program control of feedback status
	if block_settings==2		%if there is Task Program control ONLY of status (but not style)
		feedback_status=fdbk_stts_mdl;		%then use feedback status input from parent block
	elseif block_settings==3	%if there is Task Program control of both status and style
		feedback_status=4;		%then let the input VCODEs handle the status
	else						%otherwise assume that the Task Program did not provide style OR status
		feedback_status=3;		%then set both hands are always on as a default
    end
else		%if GUI is controlling feedback status
	feedback_status=fdbk_stts_GUI;
end

%set the status of the hand-feedback in the VCODES
switch feedback_status
	case 0					%show neither hand feedback
		VCODES(1,2)=0;
		VCODES(2,2)=0;
	case 1					%show ONLY dominant hand feedback
		VCODES(1,2)=1;
		VCODES(2,2)=0;
	case 2					%show ONLY non-dominant hand feedback
		VCODES(1,2)=0;
		VCODES(2,2)=1;
	case 4					%VCODES already control hand feedback
		%do nothing
	otherwise				%show both hand feedbacks
		VCODES(1,2)=1;
		VCODES(2,2)=1;
end

%----------------Feedback Position ----------------
%set the position of the hand feedback.
for i=1:2
	if i==1
		active_arm=KINARMdata(3,1);			%choose dominant arm first
	else
		active_arm=3-KINARMdata(3,1);		%choose non-dominant arm 2nd
	end
	HandXPos=KINARMdata(active_arm,23);		%(m)
	HandYPos=KINARMdata(active_arm,24);		%(m)
	HandXVel=KINARMdata(active_arm,25);		%(m/s)
	HandYVel=KINARMdata(active_arm,26);		%(m/s)

	% feed-forward hand position (m)
	HandXPos_ff = HandXPos + HandXVel*feedfwd;
	HandYPos_ff = HandYPos + HandYVel*feedfwd;
	VCODES(i,3)=HandXPos_ff;				%target position in m 
	VCODES(i,4)=HandYPos_ff;				%target position in m 
end

VCODES_out=VCODES;
